simulink model "NumSim_standard_eVTOL"  (R2024b)
settings: Solver=ode14x  StartTime=0.0  StopTime=250  FixedStep=0.005  RelTol=1e-3
values from neighbouring files (symbols this model uses):
  aDl =     [initdata.mat]
  aDr =     [initdata.mat]
  aDyn =     [initdata.mat]
  Airport = init_airport('PHNL')    [initdata_HIL_eVTOL.m]
  aLat =     [initdata.mat]
  aLon =     [initdata.mat]
  D = Prop.D    [EOM_dt_MC.m]    (also in EOM_get_alf_dt_de_prop_evtol.m = CD * QS)
  dt0 = X(2)    [EOM_get_alf_dt_de_prop_evtol.m]    (also in initdata.mat = 0.258252593971; initdata_HIL_eVTOL.m = EOM_dt_MC)
  EAS0 = TAS0 / EAS2TAS    [initdata_HIL_eVTOL.m]
  FCS = init_FCS    [initdata_HIL_eVTOL.m]
  General = init_layoutdata    [EOM_dt_MC.m]    (also in build_optimized_CA.m; initdata.mat = ; initdata_HIL_eVTOL.m)
  h0 = Con(1)    [EOM_get_alf_dt_de_prop_evtol.m]    (also in initdata.mat = 450; initdata_HIL_eVTOL.m = 50)
  mass = Con(3)    [EOM_get_alf_dt_de_prop_evtol.m]    (also in initdata.mat = 2255.54; initdata_HIL_eVTOL.m = 7)
  Motor = init_motor_evtol    [EOM_dt_MC.m]    (also in initdata.mat = []; initdata_HIL_eVTOL.m)
  Prop = init_propeller_evtol_new    [EOM_dt_MC.m]    (also in initdata_HIL_eVTOL.m)
  R2D = 180/pi    (= 57.2957795131)    [EOM_get_alf_dt_de_prop_evtol.m]    (also in init_FCS.m; init_aerodata_evtol.m; init_airport.m; initdata.mat)
  theta0 = -0.0510981441662    [initdata.mat]
undefined symbols (not defined in the file or in its folder): A1, aDa, aDe, asbhl20env, B1, C1, de0, Earth, Environment, InitData, Kd, Kp, magnitude, Tc, WGS84
libraries: simulink_extras x26, simulink x18, slpidlib x14, vrlib x8, matrix_library x6, sharedutil x6, sharedtransform x5, aerolibwindfilters x4, aerolibatmos2 x3, aerolibobsolete x2, aerolibactuator x2, aerolibasang x2
(part 2 of 7)

== system NumSim_standard_eVTOL/FCS/FCS CMD ==
  note: FlightMod
      | 1-Ready
      | 2-TakeOff
      | 3-PullUp
      | 4-Climb
      | 5-Cruise, 5.1-circle, 5.2-line
      | 6-Return
      | 7-Approach
      | 8-Flare
      | 9-TouchDown
      | 10-Taxi
      | 11-GoAround
      | 12-Parachute
  note: LonMod:
      | 1-theta hold
      | 2-height hold
      | 3-gamma control
      | 4-landing flare control
      | 5-TakeOff
  note: LatMod:
      | 1-phi hold
      | 2-lateral deviation control
      | 3-taxi y control
      | 4-
      | 5-taxi y control
  note: VMod:
      | 1-cruise throt
      | 2-max throt
      | 3-min throt
      | 4-TECS
      | 5-Flare dt Fade
  SensorData : Inport
  Land_SW : Inport  Port=2
  Bus Creator1 : BusCreator  Inputs=14
  Bus Selector : BusSelector  OutputSignals=Xe,Va,Euler
  Clock : Clock
  Divide : Product  Inputs=*/
  Divide1 : Product  Inputs=**
  Gain : Gain  Gain=-1
  Ground : Ground
  ISA Atmosphere Model : aerolibatmos2/ISA Atmosphere Model  useExtended=off  action=Warning  custom=off  viscosityOut=off  g=9.80665  gamma=1.4  R=287.0531  L=0.0065  h_trop=11000  h_strat=20000  rho0=1.225  P0=101325  T0=288.15  h0=0  S=110.4  Tref=273.15  muref=1.716e-5
  Mode Generator : Stateflow chart  TreatAsAtomicUnit=on
  Rate Limiter : RateLimiter  RisingSlewLimit=5  FallingSlewLimit=-5  SampleTimeMode=inherited
  Scope : Scope
  Selector : Selector  InputPortWidth=3  IndexOptions=Index vector (dialog)  Indices=[1]  OutputSizes=1
  Selector1 : Selector  InputPortWidth=3  IndexOptions=Index vector (dialog)  Indices=2  OutputSizes=1
  Selector2 : Selector  InputPortWidth=3  IndexOptions=Index vector (dialog)  Indices=3  OutputSizes=1
  Selector3 : Selector  InputPortWidth=3  IndexOptions=Index vector (dialog)  Indices=3  OutputSizes=1
  Sqrt : Sqrt
  Terminator : Terminator
  Terminator1 : Terminator
  Terminator2 : Terminator
  hground_value : Constant  Value=Airport.Elevation_m  OutDataTypeStr=double
  phic1 : Constant  Value=1.225
  FCSCMD : Outport  VectorParamsAs1DForOutWhenUnconnected=off
  tag scope: icmd=global
  wires:
  [V] -> Mode Generator/3(V)
  [H] -> Mode Generator/1(H)
  Clock/1 -> Mode Generator/5(time)
  Mode Generator/12(L1mod) -> Bus Creator1/12  "L1Mod"
  Mode Generator/6(Vmod) -> Bus Creator1/6  "VMod"
  Mode Generator/2(Lonmod) -> Bus Creator1/2  "LonMod"
  Mode Generator/3(thetac) -> Bus Creator1/3  "thetac"
  Mode Generator/7(Vc) -> Divide1/1, Bus Creator1/7  "Vc_EAS"
  Mode Generator/8(Latmod) -> Bus Creator1/8  "LatMod"
  Mode Generator/4(gammac) -> Bus Creator1/4  "gammac"
  Mode Generator/9(phic) -> Bus Creator1/9  "phic"
  Mode Generator/11(yc) -> Bus Creator1/11  "yc"
  Mode Generator/10(chic) -> Bus Creator1/10  "chic"
  [x] -> Mode Generator/2(x)
  SensorData/1 -> Bus Selector/1
  Bus Selector/1 -> Selector/1, Selector1/1, Selector3/1  "<Xe>"
  Selector3/1 -> Gain/1
  Selector/1 -> [x]
  Gain/1 -> [H]
  Bus Selector/2 -> [V]  "<Va>"
  Ground/1 -> Mode Generator/6(psi0)
  Bus Selector/3 -> Selector2/1  "<Euler>"
  Selector2/1 -> [psi]
  Selector1/1 -> [y]
  hground_value/1 -> Mode Generator/4(h_runway)
  Mode Generator/1(FlightMod) -> Scope/1, Bus Creator1/1  "FlightMod"
  Bus Creator1/1 -> FCSCMD/1  "FCSCMD"
  [H] -> ISA Atmosphere Model/1
  ISA Atmosphere Model/4 -> Divide/2  "rho"
  phic1/1 -> Divide/1
  Divide/1 -> Sqrt/1
  Sqrt/1 -> Divide1/2
  Divide1/1 -> Bus Creator1/13  "Vc_TAS"
  ISA Atmosphere Model/1 -> Terminator/1
  ISA Atmosphere Model/2 -> Terminator1/1
  ISA Atmosphere Model/3 -> Terminator2/1
  Land_SW/1 -> Mode Generator/7(LAND_SW)
  Mode Generator/13(icmd) -> [icmd], Bus Creator1/14  "icmd"
  Mode Generator/5(hc) -> Rate Limiter/1  "Hc"
  Rate Limiter/1 -> Bus Creator1/5  "Hc"

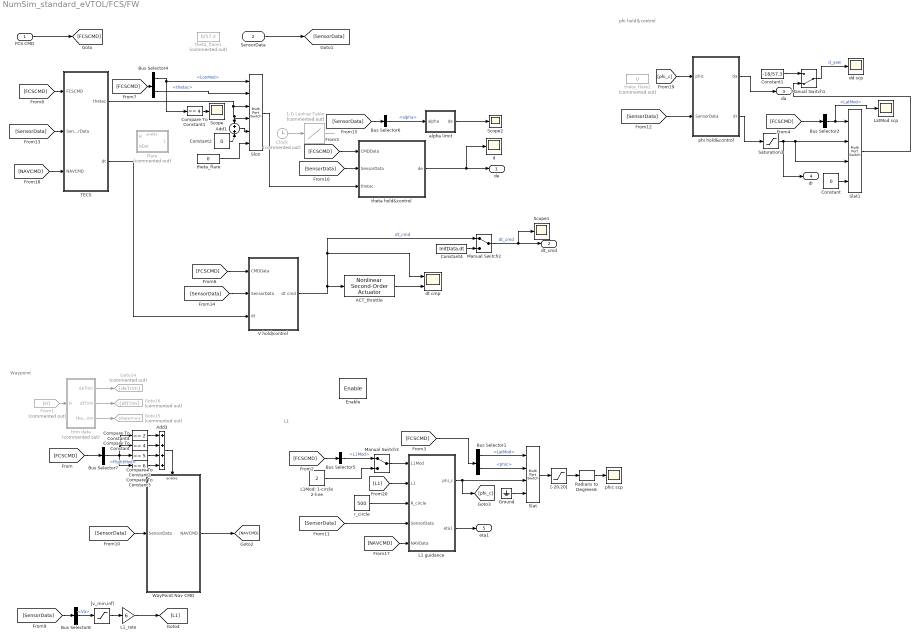
== system NumSim_standard_eVTOL/FCS/FW ==
  note: phi hold＆control
  note: L1
  note: Waypoint
  FCS CMD : Inport
  SensorData : Inport  Port=2
  Enable : EnablePort  StatesWhenEnabling=reset
  1-D Lookup Table : Lookup_n-D  Commented=on  NumberOfTableDimensions=1  BreakpointsForDimension1=[0,4,13,1e3]  Table=[-90,-90,0,0]./57.3  InternalRulePriority=Speed  RndMeth=Simplest
  ACT_throttle : aerolibactuator/Nonlinear Second-Order Actuator  wn_fin=50  z_fin=0.8  fin_max=FCS.dt_max  fin_min=FCS.dt_min  fin_maxrate=FCS.dt_rate  fin_act_0=InitData.dt  fin_act_vel=0
  Add1 : Sum  Inputs=+|+
  Add3 : Sum  Inputs=++++
  Bus Selector1 : BusSelector  OutputSignals=LatMod,phic
  Bus Selector2 : BusSelector  OutputSignals=LatMod
  Bus Selector4 : BusSelector  OutputSignals=LonMod,thetac
  Bus Selector5 : BusSelector  OutputSignals=L1Mod
  Bus Selector6 : BusSelector  OutputSignals=alpha
  Bus Selector7 : BusSelector  OutputSignals=FlightMod
  Bus Selector8 : BusSelector  OutputSignals=Va
  Clock : Clock  Commented=on
  Compare To Constant : simulink/Logic and Bit Operations/Compare To Constant  relop===  const=4  OutDataTypeStr=boolean
  Compare To Constant1 : simulink/Logic and Bit Operations/Compare To Constant  relop===  const=4  OutDataTypeStr=uint8  ZeroCross=off
  Compare To Constant2 : simulink/Logic and Bit Operations/Compare To Constant  relop===  const=5  OutDataTypeStr=boolean
  Compare To Constant3 : simulink/Logic and Bit Operations/Compare To Constant  relop===  const=6  OutDataTypeStr=boolean
  Compare To Constant4 : simulink/Logic and Bit Operations/Compare To Constant  relop===  const=2  OutDataTypeStr=boolean
  Constant : Constant  Value=0
  Constant1 : Constant  Value=-18/57.3
  Constant2 : Constant  Value=0
  Constant4 : Constant  Value=InitData.dt
  Flare : Subsystem  Commented=on
  From1 : From  Commented=on  GotoTag=H
      settings: CloseFcn=tagdialog Close
  Goto14 : Goto  Commented=on  GotoTag=deTrim  TagVisibility=scoped
  Goto15 : Goto  Commented=on  GotoTag=thetaTrim  TagVisibility=scoped
  Goto16 : Goto  Commented=on  GotoTag=dtTrim  TagVisibility=scoped
  Ground : Ground
  L1 guidance : Subsystem  RequirementInfo={} %GIDa_679a8677_8221_4c9e_b86c_be3e68c5d594
  L1Mod: 1-circle 2-line : Constant  Value=2
  L1_rate : Gain  Gain=6
  LatMod scp : Scope
  Manual Switch1 : ManualSwitch  CurrentSetting=0
  Manual Switch2 : ManualSwitch
  Manual Switch3 : ManualSwitch
  Radians to Degrees6 : simulink_extras/Transformations/Radians to Degrees
  Saturation3 : Saturate  UpperLimit=0.3  LowerLimit=-0.3
  Scope : Scope
  Scope1 : Scope
  Scope2 : Scope
  Slat : MultiPortSwitch  SaturateOnIntegerOverflow=off  InputSameDT=off
  Slat1 : MultiPortSwitch  SaturateOnIntegerOverflow=off  InputSameDT=off
  Slon : MultiPortSwitch  Inputs=5  DataPortIndices={2}  SaturateOnIntegerOverflow=off  InputSameDT=off
  TECS : Subsystem
  V hold/control : Subsystem
  WayPoint Nav CMD : Subsystem
  "[-20,20]" : Saturate  UpperLimit=20*pi/180  LowerLimit=-20*pi/180
  "[v_min,inf)" : Saturate  UpperLimit=inf  LowerLimit=FCS.V_min
  alpha limit : Subsystem
  d : Scope
  dd scp : Scope
  dt cmp : Scope  NumInputPorts=2
  phi hold&control : Subsystem
  phic scp : Scope
  r_circle : Constant  Value=500
  theta hold&control : Subsystem
  theta_flare : Constant  Value=0
  theta_flare1 : Constant  Commented=on  Value=0/57.3
  theta_flare2 : Constant  Commented=on  Value=0
  trim data : Subsystem  Commented=on
  de : Outport
  dt_cmd : Outport  Port=2
  da : Outport  Port=3
  dr : Outport  Port=4
  eta1 : Outport  Port=5
  wires:
  Compare To Constant4/1 -> Add3/1
  Bus Selector1/1 -> Slat/1  "<LatMod>"
  trim data/1(deTrim) -> Goto14/1
  WayPoint Nav CMD/1(NAVCMD) -> [NAVCMD]
  L1 guidance/2(eta1) -> eta1/1
  Slat/1 -> "[-20,20]"/1
  "[-20,20]"/1 -> Radians to Degrees6/1
  Add3/1 -> WayPoint Nav CMD/Enable
  r_circle/1 -> L1 guidance/3(R_circle)
  alpha limit/1(de) -> Scope2/1
  Ground/1 -> Slat/4
  V hold/control/1(dt cmd) -> Manual Switch2/1, dt cmp/1, ACT_throttle/1  "dt_cmd"
  L1Mod: 1-circle 2-line/1 -> Manual Switch3/2
  Constant4/1 -> Manual Switch2/2
  trim data/3(thetaTrim) -> Goto15/1
  ACT_throttle/1 -> dt cmp/2
  SensorData/1 -> [SensorData]
  Slat1/1 -> Manual Switch1/2
  Manual Switch1/1 -> dd scp/1  "d_yaw"
  Add1/1 -> Slon/5
  theta_flare/1 -> Slon/6
  Bus Selector2/1 -> LatMod scp/1, Slat1/1  "<LatMod>"
  Bus Selector5/1 -> Manual Switch3/1  "<L1Mod>"
  Bus Selector6/1 -> alpha limit/1(alpha)  "<alpha>"
  Bus Selector7/1 -> Compare To Constant3/1, Compare To Constant4/1, Compare To Constant/1, Compare To Constant2/1  "<FlightMod>"
  "[v_min,inf)"/1 -> L1_rate/1
  Clock/1 -> 1-D Lookup Table/1
  TECS/1(thetac) -> Add1/1, Slon/4, Slon/3
  Saturation3/1 -> dr/1, Slat1/3, Slat1/2
  Slon/1 -> theta hold&control/3(thetac)
  Bus Selector4/1 -> Compare To Constant1/1, Slon/1  "<LonMod>"
  1-D Lookup Table/1 -> ?
  TECS/2(dt) -> V hold/control/3(dt)
  Radians to Degrees6/1 -> phic scp/1
  Bus Selector4/2 -> Slon/2  "<thetac>"
  Bus Selector8/1 -> "[v_min,inf)"/1  "<Va>"
  From1/1 -> trim data/1(H)
  Manual Switch3/1 -> L1 guidance/1(L1Mod)
  phi hold&control/2(dr) -> Saturation3/1
  FCS CMD/1 -> [FCSCMD]
  Compare To Constant2/1 -> Add3/3
  Manual Switch2/1 -> Scope1/1, dt_cmd/1  "dt_cmd"
  Constant1/1 -> Manual Switch1/1
  Compare To Constant3/1 -> Add3/4
  trim data/2(dtTrim) -> Goto16/1
  Compare To Constant/1 -> Add3/2
  Bus Selector1/2 -> Slat/2  "<phic>"
  Constant2/1 -> Add1/2
  Constant/1 -> Slat1/4
  Compare To Constant1/1 -> Scope/1
  L1 guidance/1(phi_c) -> [phi_c], Slat/3
  theta hold&control/1(de) -> d/1, de/1
  phi hold&control/1(da) -> da/1
  [FCSCMD] -> Bus Selector7/1
  [FCSCMD] -> Bus Selector5/1
  [FCSCMD] -> Bus Selector1/1
  [FCSCMD] -> Bus Selector2/1
  [FCSCMD] -> theta hold&control/1(CMDData)
  [FCSCMD] -> V hold/control/1(CMDData)
  [FCSCMD] -> Bus Selector4/1
  [FCSCMD] -> TECS/1(FCSCMD)
  [SensorData] -> Bus Selector8/1
  [SensorData] -> WayPoint Nav CMD/1(SensorData)
  [SensorData] -> L1 guidance/4(SensorData)
  [SensorData] -> phi hold&control/2(SensorData)
  [SensorData] -> TECS/2(SensorData)
  [SensorData] -> V hold/control/2(SensorData)
  [SensorData] -> Bus Selector6/1
  [SensorData] -> theta hold&control/2(SensorData)
  [NAVCMD] -> L1 guidance/5(NAVData)
  [NAVCMD] -> TECS/3(NAVCMD)
  [phi_c] -> phi hold&control/1(phic)
  L1_rate/1 -> [L1]
  [L1] -> L1 guidance/2(L1)

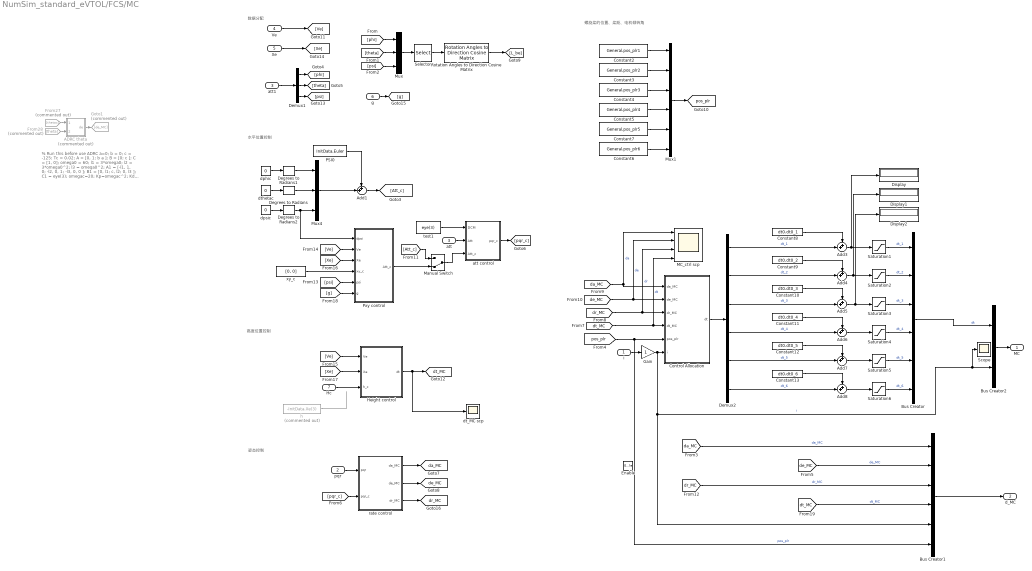
== system NumSim_standard_eVTOL/FCS/MC ==
  note: 数据分配
  note: 螺旋桨的位置、桨距、电机倾转角
  note: 姿态控制
  note: 高度位置控制
  note: 水平位置控制
  note: % Run this before use ADRC
      | a=0;
      | b = 0;
      | c = -125;
      | Tc = 0.02;
      | A = [0, 1; b a ];
      | B = [0; c ];
      | C = [1, 0];
      | omega0 = 60;
      | l1 = 3*omega0;
      | l2 = 3*omega0^2;
      | l3 = omega0^2;
      | A1 = [-l1,  1,  0; -l2,  0,  1; -l3,  0,  0 ];
      | B1 = [0,  l1; c,  l2; 0,  l3 ];
      | C1 = eye(3);
      | omegac=20;
      | Kp=omegac^2;
      | Kd = 2*omegac;
  i : Inport
  pqr : Inport  Port=2
  att : Inport  Port=3
  Ve : Inport  Port=4
  Xe : Inport  Port=5
  g : Inport  Port=6
  Hc : Inport  Port=7
  Enable : EnablePort  StatesWhenEnabling=reset
  ADRC theta : Subsystem  Commented=on
  Add{1,3..8} (7 alike) : Sum  Inputs=++|
  Bus Creator : BusCreator  Inputs=6
  Bus Creator1 : BusCreator  Inputs=6
  Bus Creator2 : BusCreator  Inputs=2
  Constant10 : Constant  Value=dt0.dt0_3
  Constant11 : Constant  Value=dt0.dt0_4
  Constant12 : Constant  Value=dt0.dt0_5
  Constant13 : Constant  Value=dt0.dt0_6
  Constant2 : Constant  Value=General.pos_plr1
  Constant3 : Constant  Value=General.pos_plr2
  Constant4 : Constant  Value=General.pos_plr3
  Constant5 : Constant  Value=General.pos_plr4
  Constant6 : Constant  Value=General.pos_plr6
  Constant7 : Constant  Value=General.pos_plr5
  Constant8 : Constant  Value=dt0.dt0_1
  Constant9 : Constant  Value=dt0.dt0_2
  Control Allocation : MATLAB Function  TreatAsAtomicUnit=on
  Degrees to Radians : simulink_extras/Transformations/Degrees to Radians
  Degrees to Radians1 : simulink_extras/Transformations/Degrees to Radians
  Degrees to Radians2 : simulink_extras/Transformations/Degrees to Radians
  Demux1 : Demux  Outputs=3
  Demux2 : Demux  Outputs=6
  Display : Display
  Display1 : Display
  Display2 : Display
  From27 : From  Commented=on  GotoTag=thetac
  From28 : From  Commented=on  GotoTag=theta
  Gain : Gain
  Goto1 : Goto  Commented=on  GotoTag=de_MC
  Height control : Subsystem
  MC_ctrl scp : Scope  NumInputPorts=4
  Manual Switch : ManualSwitch  CurrentSetting=0
  Mux : Mux  Inputs=3
  Mux1 : Mux  Inputs=6
  Mux4 : Mux  Inputs=3
  PSI0 : Constant  Value=InitData.Euler
  Pxy control : Subsystem
  Rotation Angles to Direction Cosine Matrix : sharedtransform/Rotation Angles to Direction Cosine Matrix  rotationOrder=ZYX  aMode=aMode
  Saturation{1..6} (6 alike) : Saturate  UpperLimit=1  LowerLimit=0
  Scope : Scope
  Selector : Selector  InputPortWidth=3  IndexOptions=Index vector (dialog)  Indices=[3,2,1]  OutputSizes=1
  att control : Subsystem
  att1 : InportShadow  Port=3
  dphic : Constant  Value=0
  dpsic : Constant  Value=0
  dt_MC scp : Scope
  dthetac : Constant  Value=0
  h : Constant  Commented=on  Value=-InitData.Xe(3)
  rate control : Subsystem
  test1 : Constant  Value=eye(3)
  xy_c : Constant  Value=[0, 0]
  MC : Outport
  d_MC : Outport  Port=2
  tag scope: da_MC=global, de_MC=global, dr_MC=global, dt_MC=global, pos_plr=global
  wires:
  Demux2/3 -> Add5/2  "dt_3"
  Demux2/2 -> Add4/2  "dt_2"
  Demux2/4 -> Add6/2  "dt_4"
  Demux2/1 -> Add3/2  "dt_1"
  Bus Creator/1 -> Bus Creator2/1  "dt"
  Rotation Angles to Direction Cosine Matrix/1 -> [L_be]
  Mux/1 -> Selector/1
  Selector/1 -> Rotation Angles to Direction Cosine Matrix/1
  [phi] -> Mux/1
  [psi] -> Mux/3
  Degrees to Radians/1 -> Mux4/2
  Degrees to Radians2/1 -> Pxy control/1(dpsi), Mux4/3
  [theta] -> Mux/2
  dphic/1 -> Degrees to Radians1/1
  dpsic/1 -> Degrees to Radians2/1
  Degrees to Radians1/1 -> Mux4/1
  [dt_MC] -> MC_ctrl scp/4, Control Allocation/4(dt_MC)  "dt"
  [da_MC] -> MC_ctrl scp/1, Control Allocation/1(da_MC)  "da"
  [de_MC] -> MC_ctrl scp/2, Control Allocation/2(de_MC)  "de"
  [dr_MC] -> MC_ctrl scp/3, Control Allocation/3(dr_MC)  "dr"
  From28/1 -> ADRC theta/2(theta)
  ADRC theta/1(de) -> Goto1/1
  From27/1 -> ADRC theta/1(thetac)
  pqr/1 -> rate control/1(pqr)
  [pqr_c] -> rate control/2(pqr_c)
  att/1 -> att control/2(Att)
  att control/1(pqr_c) -> [pqr_c]
  Mux4/1 -> Add1/2
  [Att_c] -> Manual Switch/1
  att1/1 -> Demux1/1
  Demux1/1 -> [phi]
  Demux1/3 -> [psi]
  Demux1/2 -> [theta]
  Ve/1 -> [Ve]
  Xe/1 -> [Xe]
  Pxy control/1(Att_c) -> Manual Switch/2
  xy_c/1 -> Pxy control/4(xy_c)
  Manual Switch/1 -> att control/3(Att_c)
  Add1/1 -> [Att_c]
  PSI0/1 -> Add1/1
  Control Allocation/1(dt) -> Demux2/1
  Height control/1(dt) -> dt_MC scp/1, [dt_MC]
  test1/1 -> att control/1(DCM)
  Hc/1 -> Height control/3(h_c)
  h/1 -> ?
  dthetac/1 -> Degrees to Radians/1
  Demux2/5 -> Add7/2  "dt_5"
  Demux2/6 -> Add8/2  "dt_6"
  rate control/1(da_MC) -> [da_MC]
  rate control/2(de_MC) -> [de_MC]
  rate control/3(dr_MC) -> [dr_MC]
  Constant2/1 -> Mux1/1
  Constant3/1 -> Mux1/2
  Constant4/1 -> Mux1/3
  Constant5/1 -> Mux1/4
  Constant7/1 -> Mux1/5
  Constant6/1 -> Mux1/6
  Mux1/1 -> [pos_plr]
  [pos_plr] -> Bus Creator1/6, Control Allocation/5(pos_plr)  "pos_plr"
  Gain/1 -> Scope/1, Bus Creator2/2, Bus Creator1/5, Control Allocation/6(i)  "i"
  Bus Creator2/1 -> MC/1
  Saturation1/1 -> Bus Creator/1  "dt_1"
  Saturation2/1 -> Bus Creator/2  "dt_2"
  Saturation3/1 -> Bus Creator/3  "dt_3"
  Saturation4/1 -> Bus Creator/4  "dt_4"
  Saturation5/1 -> Bus Creator/5  "dt_5"
  Saturation6/1 -> Bus Creator/6  "dt_6"
  Constant8/1 -> Add3/1
  Add3/1 -> Display/1, Saturation1/1
  Constant9/1 -> Add4/1
  Add4/1 -> Display1/1, Saturation2/1
  Constant10/1 -> Add5/1
  Add5/1 -> Display2/1, Saturation3/1
  Constant11/1 -> Add6/1
  Add6/1 -> Saturation4/1
  Constant12/1 -> Add7/1
  Add7/1 -> Saturation5/1
  Constant13/1 -> Add8/1
  Add8/1 -> Saturation6/1
  [psi] -> Pxy control/5(psi)
  [Ve] -> Pxy control/2(Ve)
  [Ve] -> Height control/1(Ve)
  [Xe] -> Pxy control/3(Xe)
  [Xe] -> Height control/2(Xe)
  g/1 -> [g]
  [g] -> Pxy control/6(g)
  i/1 -> Gain/1
  [de_MC] -> Bus Creator1/2  "de_MC"
  [dt_MC] -> Bus Creator1/4  "dt_MC"
  Bus Creator1/1 -> d_MC/1
  [da_MC] -> Bus Creator1/1  "da_MC"
  [dr_MC] -> Bus Creator1/3  "dr_MC"

== system NumSim_standard_eVTOL/FCS/control selector ==
  note: CtrlMod:
      | 1-pqr control
      | 2-att control
      | 3-path angle control
      | 4-way point control
      | 5-TakeOff
      | 6-Parachute land
  note: FlightStage
      | 1-Ready
      | 2-TakeOff
      | 3-PullUp
      | 4-Climb
      | 5-Cruise, 5.1-circle, 5.2-line
      | 6-Return
      | 7-Approach
      | 8-Flare
      | 9-TouchDown
      | 10-Taxi
      | 11-GoAround
      | 12-Parachute
  Bus Selector1 : BusSelector  Commented=on  OutputSignals=FlightMod
  Constant1 : Constant  Commented=on
  Constant8 : Constant  Commented=on  Value=0
  Constant9 : Constant  Commented=on
  From1 : From  Commented=on  GotoTag=CutAct
  From2 : From  Commented=on  GotoTag=CutAct
  From3 : From  Commented=on  GotoTag=CutAct
  From9 : From  Commented=on  GotoTag=deTrim  TagVisibility=scoped
      settings: CloseFcn=tagdialog Close
  Goto5 : Goto  Commented=on  GotoTag=CutAct
  Merge : Merge  Commented=on
  Product{,1..3} (4 alike) : Product  Commented=on
  Radians to Degrees1 : simulink_extras/Transformations/Radians to Degrees  Commented=on
  Scope : Scope  Commented=on
  Scope1 : Scope  Commented=on
  Switch Case : SwitchCase  Commented=on  CaseConditions={[2,12]}
  Switch Case Action Subsystem1 : Subsystem  Commented=on  TreatAsAtomicUnit=on
  Switch Case Action Subsystem2 : Subsystem  Commented=on  TreatAsAtomicUnit=on
  dr scp : Scope  Commented=on
  dt scp : Scope  Commented=on
  wires:
  Product/1 -> dt scp/1
  Switch Case Action Subsystem2/1(Out1) -> Merge/1
  Constant9/1 -> Switch Case Action Subsystem1/1(In1)  "keep"
  Switch Case Action Subsystem1/1(Out1) -> Merge/2
  Switch Case/1 -> Switch Case Action Subsystem2/Action
  Bus Selector1/1 -> Scope1/1, Switch Case/1  "<FlightMod>"
  Switch Case/2 -> Switch Case Action Subsystem1/Action
  Constant8/1 -> Switch Case Action Subsystem2/1(In1)  "cut"
  Merge/1 -> Goto5/1
  Constant1/1 -> Product/1
  From1/1 -> Product1/2
  From3/1 -> Product3/2
  From2/1 -> Product2/2
  Product2/1 -> dr scp/1
  Product1/1 -> Radians to Degrees1/1
  Radians to Degrees1/1 -> Scope/1
  ? -> ?

== system NumSim_standard_eVTOL/airframe/Flight Conditions ==
  EnvmData : Inport
  PlantData : Inport  Port=2
  Bus Selector1 : BusSelector  OutputSignals=WindVelocity,a,AirDensity,WindAngularRates,Po,To,g
  Bus Selector2 : BusSelector  OutputSignals=Ve,Vb,pqr,DCM_be
  Derivative : Derivative  CoefficientInTFapproximation=100
  Dynamic Pressure : aerolibasang/Dynamic Pressure
  "Incidence, Sideslip, & Airspeed" : Subsystem  AncestorBlock=aerolibasang/Incidence, Sideslip, & Airspeed  mask(Incidence,Sideslip,&Airspeed){}
      mask help: Calculate the angles between the body and the velocity vector (incidence and sideslip), and the velocity magnitude from the components in body axes (Vb).
      settings: LibrarySourceBlock=|
      | aerolibasang/Incidence, Sideslip,
      | & Airspeed
      mask Help: web(asbhelp('incidence'));
      mask Display:
      | port_label('input',1,'V_b','texmode','on');
      | port_label('output',1,'\alpha','texmode','on');
      | port_label('output',2,'\beta','texmode','on');
      | port_label('output',3,'V','texmode','on');
  Mach Number : aerolibasang/Mach Number
  Product : Product  Multiplication=Matrix(*)
  Product1 : Product  Multiplication=Matrix(*)
  Subsystem : Subsystem
  Sum1 : Sum  Inputs=+-|  InputSameDT=on  SaturateOnIntegerOverflow=on  OutDataTypeStr=Inherit: Same as first input
  Sum2 : Sum  Inputs=|+-  InputSameDT=on  SaturateOnIntegerOverflow=on  OutDataTypeStr=Inherit: Same as first input
  Terminator : Terminator
  Va_b : Scope
  Vk_b : Scope
  Vw_b : Scope
  Vw_e : Scope
  Alpha : Outport  VectorParamsAs1DForOutWhenUnconnected=off
  AlphaDot : Outport  Port=2  VectorParamsAs1DForOutWhenUnconnected=off
  Beta : Outport  Port=3  VectorParamsAs1DForOutWhenUnconnected=off
  V : Outport  Port=4  VectorParamsAs1DForOutWhenUnconnected=off
  pqrWind : Outport  Port=5  VectorParamsAs1DForOutWhenUnconnected=off
  Mach : Outport  Port=6  VectorParamsAs1DForOutWhenUnconnected=off
  Qbar : Outport  Port=7  InitialOutput=0  VectorParamsAs1DForOutWhenUnconnected=off
  gamma : Outport  Port=8  InitialOutput=0  VectorParamsAs1DForOutWhenUnconnected=off
  chi : Outport  Port=9  InitialOutput=0  VectorParamsAs1DForOutWhenUnconnected=off
  Po : Outport  Port=10  VectorParamsAs1DForOutWhenUnconnected=off
  To : Outport  Port=11  VectorParamsAs1DForOutWhenUnconnected=off
  g : Outport  Port=12  VectorParamsAs1DForOutWhenUnconnected=off
  wires:
  Derivative/1 -> AlphaDot/1
  Bus Selector1/4 -> Product1/2  "<WindAngularRates>"
  Subsystem/1(gamma) -> gamma/1
  PlantData/1 -> Bus Selector2/1
  Sum2/1 -> "Incidence, Sideslip, & Airspeed"/1(Vb), Va_b/1, Mach Number/1, Dynamic Pressure/1  "VA(b)"
  Subsystem/2(chi) -> chi/1
  Bus Selector2/2 -> Vk_b/1, Sum2/1  "<Vb>"
  Subsystem/3(V) -> Terminator/1
  Product1/1 -> Sum1/2
  Bus Selector1/5 -> Po/1  "<Po>"
  Mach Number/1 -> Mach/1  "Mach"
  "Incidence, Sideslip, & Airspeed"/1(Alpha) -> Derivative/1, Alpha/1  "Alpha"
  Product/1 -> Vw_b/1, Sum2/2
  Bus Selector2/1 -> Subsystem/1(<Ve>)  "<Ve>"
  "Incidence, Sideslip, & Airspeed"/2(Beta) -> Beta/1  "Beta"
  "Incidence, Sideslip, & Airspeed"/3(V) -> V/1  "V"
  Dynamic Pressure/1 -> Qbar/1  "qbar"
  Bus Selector1/2 -> Mach Number/2  "<a>"
  Bus Selector2/4 -> Product/1, Product1/1  "<DCM_be>"
  Bus Selector2/3 -> Sum1/1  "<pqr>"
  Sum1/1 -> pqrWind/1
  EnvmData/1 -> Bus Selector1/1
  Bus Selector1/3 -> Dynamic Pressure/2  "<AirDensity>"
  Bus Selector1/1 -> Product/2, Vw_e/1  "<WindVelocity>"
  Bus Selector1/7 -> g/1  "<g>"
  Bus Selector1/6 -> To/1  "<To>"

== system NumSim_standard_eVTOL/airframe/force moment ==
  note: force and moment in body fixed axis coordination
  PlantData : Inport
  Act_surface : Inport  Port=2
  prop : Inport  Port=3
  EnvmData : Inport  Port=4
  Add : Sum  Inputs=++++
  Add1 : Sum  Inputs=++++
  Disturbance : Constant  Value=[0,10,0]
  Disturbance1 : Constant  Value=[0,0,0]
  F_Gear_in_b scp : Scope  Commented=on
  Gear&FM in body axis : Subsystem  Commented=on
  M_Gear scp : Scope  Commented=on
  Manual Switch : ManualSwitch  CurrentSetting=0
  Motor moment scp : Scope
  Scope{,1..4,6} (6 alike) : Scope
  Thrust&M in body axis : Subsystem
  aero F&M in body axis : Subsystem
  gravity in body axis : Subsystem
  Fb (X Y Z) : Outport  VectorParamsAs1DForOutWhenUnconnected=off
  M (L M N) : Outport  Port=2  VectorParamsAs1DForOutWhenUnconnected=off
  wires:
  Thrust&M in body axis/1(f_T) -> Add/1, Scope4/1
  gravity in body axis/1(Fb) -> Add/3, Scope3/1
  Thrust&M in body axis/2(m_T) -> Add1/1, Motor moment scp/1
  aero F&M in body axis/2(M (L M N)) -> Scope6/1, Add1/2
  Add1/1 -> Scope1/1, M (L M N)/1
  Add/1 -> Scope/1, Fb (X Y Z)/1
  PlantData/1 -> aero F&M in body axis/1(PlantData), Gear&FM in body axis/1(PlantData), gravity in body axis/1(PlantData)
  Act_surface/1 -> aero F&M in body axis/2(Act_surface)
  EnvmData/1 -> gravity in body axis/2(EnvmData)
  Gear&FM in body axis/1(F_Gear) -> Add/4, F_Gear_in_b scp/1
  Gear&FM in body axis/2(M_Gear) -> Add1/3, M_Gear scp/1
  aero F&M in body axis/1(Fb (X Y Z)) -> Add/2, Scope2/1
  Disturbance/1 -> Manual Switch/1
  Manual Switch/1 -> Add1/4
  Disturbance1/1 -> Manual Switch/2
  prop/1 -> Thrust&M in body axis/1(prop)

== system NumSim_standard_eVTOL/Energy & Power/V_prop1/v_b to v_prop ==
  V_body : Inport
  i : Inport  Port=2
  Add : Sum  Inputs=+-
  Mux1 : Mux  Inputs=2
  Terminator : Terminator
  V_x : Fcn  Expr=u[1]*cos(u[4])
  V_y : Fcn  Expr=0
  V_z : Fcn  Expr=u[3]*sin(u[4])
  V : Outport  VectorParamsAs1DForOutWhenUnconnected=off
  wires:
  i/1 -> Mux1/2
  V_body/1 -> Mux1/1
  Mux1/1 -> V_z/1, V_y/1, V_x/1
  Add/1 -> V/1
  V_x/1 -> Add/1
  V_z/1 -> Add/2
  V_y/1 -> Terminator/1

== system NumSim_standard_eVTOL/Energy & Power/V_prop2/v_b to v_prop ==
  V_body : Inport
  i : Inport  Port=2
  Add : Sum  Inputs=+-
  Mux1 : Mux  Inputs=2
  Terminator : Terminator
  V_x : Fcn  Expr=u[1]*cos(u[4])
  V_y : Fcn  Expr=0
  V_z : Fcn  Expr=u[3]*sin(u[4])
  V : Outport  VectorParamsAs1DForOutWhenUnconnected=off
  wires:
  i/1 -> Mux1/2
  V_body/1 -> Mux1/1
  Mux1/1 -> V_z/1, V_y/1, V_x/1
  V_z/1 -> Add/2
  V_x/1 -> Add/1
  Add/1 -> V/1
  V_y/1 -> Terminator/1

== system NumSim_standard_eVTOL/Energy & Power/V_prop3/v_b to v_prop ==
  V_body : Inport
  i : Inport  Port=2
  Add : Sum  Inputs=+-
  Mux1 : Mux  Inputs=2
  Terminator : Terminator
  V_x : Fcn  Expr=u[1]*cos(u[4])
  V_y : Fcn  Expr=0
  V_z : Fcn  Expr=u[3]*sin(u[4])
  V : Outport  VectorParamsAs1DForOutWhenUnconnected=off
  wires:
  i/1 -> Mux1/2
  V_body/1 -> Mux1/1
  Mux1/1 -> V_z/1, V_y/1, V_x/1
  V_z/1 -> Add/2
  V_x/1 -> Add/1
  Add/1 -> V/1
  V_y/1 -> Terminator/1

== system NumSim_standard_eVTOL/Energy & Power/V_prop4/v_b to v_prop ==
  V_body : Inport
  i : Inport  Port=2
  Add : Sum  Inputs=+-
  Mux1 : Mux  Inputs=2
  Terminator : Terminator
  V_x : Fcn  Expr=u[1]*cos(u[4])
  V_y : Fcn  Expr=0
  V_z : Fcn  Expr=u[3]*sin(u[4])
  V : Outport  VectorParamsAs1DForOutWhenUnconnected=off
  wires:
  i/1 -> Mux1/2
  V_body/1 -> Mux1/1
  Mux1/1 -> V_z/1, V_y/1, V_x/1
  V_x/1 -> Add/1
  Add/1 -> V/1
  V_z/1 -> Add/2
  V_y/1 -> Terminator/1

== system NumSim_standard_eVTOL/Energy & Power/V_prop5/v_b to v_prop ==
  V_body : Inport
  i : Inport  Port=2
  Add : Sum  Inputs=+-
  Mux1 : Mux  Inputs=2
  Terminator : Terminator
  V_x : Fcn  Expr=u[1]*cos(u[4])
  V_y : Fcn  Expr=0
  V_z : Fcn  Expr=u[3]*sin(u[4])
  V : Outport  VectorParamsAs1DForOutWhenUnconnected=off
  wires:
  i/1 -> Mux1/2
  V_body/1 -> Mux1/1
  Mux1/1 -> V_z/1, V_y/1, V_x/1
  V_z/1 -> Add/2
  V_x/1 -> Add/1
  Add/1 -> V/1
  V_y/1 -> Terminator/1

== system NumSim_standard_eVTOL/Energy & Power/V_prop6/v_b to v_prop ==
  V_body : Inport
  i : Inport  Port=2
  Add : Sum  Inputs=+-
  Mux1 : Mux  Inputs=2
  Terminator : Terminator
  V_x : Fcn  Expr=u[1]*cos(u[4])
  V_y : Fcn  Expr=0
  V_z : Fcn  Expr=u[3]*sin(u[4])
  V : Outport  VectorParamsAs1DForOutWhenUnconnected=off
  wires:
  i/1 -> Mux1/2
  V_body/1 -> Mux1/1
  Mux1/1 -> V_z/1, V_y/1, V_x/1
  V_z/1 -> Add/2
  V_x/1 -> Add/1
  Add/1 -> V/1
  V_y/1 -> Terminator/1

== system NumSim_standard_eVTOL/Energy & Power/thrust_1/Motor ==
  P_shaft : Inport
  dt : Inport  Port=2
  V : Inport  Port=3
  rpm0 : Inport  Port=4
  rho : Inport  Port=5
  rpm_grid : Inport  Port=6
  Add : Sum
  Constant : Constant  Value=Motor.Ue
  Constant1 : Constant  Value=Motor.Re
  Constant2 : Constant  Value=Motor.Rm
  Constant3 : Constant  Value=Motor.KE
  Constant4 : Constant  Value=Motor.KT  VectorParams1D=off
  Constant5 : Constant  Value=Motor.Im0
  Constant6 : Constant  Value=0
  Constant7 : Constant  Value=0.001
  D^5 : Constant  Value=5
  Diameter : Constant  Value=Prop.D
  Diameter1 : Constant  Value=Prop.D
  Divide : Product  Inputs=*//
  Ea : Sum  Inputs=+-
  Gain1 : Gain  Gain=30/pi
  Gain2 : Gain  Gain=pi/30
  Gain3 : Gain  Gain=1/60
  Gain4 : Gain  Gain=1/(2*pi)
  Im : Sum
  Integrator : Integrator  InitialConditionSource=external  InitialCondition=600
  Ix : Constant  Value=Prop.Ix
  J : Product  Inputs=*//
  Manual Switch : ManualSwitch
  Math Function : Math  Operator=magnitude^2  SignedPower=on
  Math Function3 : Math  Operator=pow  SignedPower=on
  Math Function4 : Math  Operator=pow  SignedPower=on
  Memory : Memory  InitialCondition=0.1
  N(rpm) : Product  Inputs=*/
  N(rpm)1 : Product  Inputs=/*
  P Scope : Scope  NumInputPorts=2
  P_sp : Product  Inputs=4
  Product1 : Product
  Product2 : Product
  Q : Product  Inputs=4
  RPM 1 : Scope  NumInputPorts=2
  Saturation : Saturate  UpperLimit=1047.2  LowerLimit=0.1
  Scope : Scope
  Sum : Sum  Inputs=|+-
  Ueo : Product
  Um : Sum  Inputs=+-
  get CP : Lookup_n-D  BreakpointsForDimension1=Prop.J  BreakpointsForDimension2=Prop.rpm_grid  IndexSearchMethod=Linear search  BeginIndexSearchUsingPreviousIndexResult=on  Table=Prop.CP  RndMeth=Simplest
      settings: InputPortMap=u0,u1
  "n^3 " : Constant  Value=3
  rpm : Outport  VectorParamsAs1DForOutWhenUnconnected=off
  wires:
  Saturation/1 -> Gain1/1, Divide/2
  Gain2/1 -> Integrator/2
  rpm0/1 -> Manual Switch/1
  Gain1/1 -> rpm/1, RPM 1/1  "rpm"
  Sum/1 -> Divide/1  "DP"
  Divide/1 -> Integrator/1  "omega_dot"
  Integrator/1 -> Saturation/1  "omega"
  P_sp/1 -> Scope/1, P Scope/1, Sum/1
  P_shaft/1 -> P Scope/2, Sum/2
  Ix/1 -> Divide/3
  Constant/1 -> Ueo/2
  Ueo/1 -> Um/1
  Product1/1 -> Um/2
  Constant1/1 -> Product1/1
  Um/1 -> Ea/1
  Product2/1 -> Ea/2
  Constant2/1 -> Product2/1
  Ea/1 -> N(rpm)/1
  Constant3/1 -> N(rpm)/2
  Diameter/1 -> J/2
  V/1 -> J/1
  N(rpm)/1 -> Gain3/1, RPM 1/2
  J/1 -> get CP/1
  Gain4/1 -> Q/2  "CQ"
  D^5/1 -> Math Function4/2
  Diameter1/1 -> Math Function4/1
  Math Function/1 -> Q/3  "n^2"
  Q/1 -> N(rpm)1/2
  Constant4/1 -> N(rpm)1/1
  N(rpm)1/1 -> Im/1
  Constant5/1 -> Im/2
  Im/1 -> Product2/2, Product1/2
  rho/1 -> Q/1, P_sp/3  "rho"
  Math Function3/1 -> P_sp/2  "n^3"
  "n^3 "/1 -> Math Function3/2
  Math Function4/1 -> Q/4, P_sp/4  "D^5"
  get CP/1 -> P_sp/1, Gain4/1  "CP"
  Manual Switch/1 -> Gain2/1
  Constant6/1 -> Manual Switch/2
  Constant7/1 -> Add/1
  Add/1 -> Ueo/1
  dt/1 -> Add/2
  Gain3/1 -> Memory/1  "rps"
  Memory/1 -> J/3, Math Function3/1, Math Function/1
  rpm_grid/1 -> get CP/2

== system NumSim_standard_eVTOL/Energy & Power/thrust_1/Propeller  ==
  rpm : Inport
  V : Inport  Port=2
  rho : Inport  Port=3
  D^5 : Constant  Value=5
  Diameter : Constant  Value=Prop.D
  Display1 : Display
  Display7 : Display
  Divide : Product  Inputs=4
  Divide2 : Product  Inputs=4
  Divide3 : Product  Inputs=**/
  Gain : Gain  Gain=1/60
  Math Function : Math  Operator=magnitude^2  SignedPower=on
  Math Function1 : Math  Operator=magnitude^2  SignedPower=on
  Math Function2 : Math  Operator=magnitude^2  SignedPower=on
  Math Function3 : Math  Operator=pow  SignedPower=on
  Math Function4 : Math  Operator=pow  SignedPower=on
  Scope{,1..4} (5 alike) : Scope
  Subsystem : Subsystem
  get CP : Lookup_n-D  BreakpointsForDimension1=Prop.J  BreakpointsForDimension2=Prop.rpm_grid  IndexSearchMethod=Linear search  BeginIndexSearchUsingPreviousIndexResult=on  Table=Prop.CP  RndMeth=Simplest
      settings: InputPortMap=u0,u1
  get CT : Lookup_n-D  BreakpointsForDimension1=Prop.J  BreakpointsForDimension2=Prop.rpm_grid  IndexSearchMethod=Linear search  BeginIndexSearchUsingPreviousIndexResult=on  Table=Prop.CT  RndMeth=Simplest
      settings: InputPortMap=u0,u1
  "n^3 " : Constant  Value=3
  P_plr (w) : Outport  VectorParamsAs1DForOutWhenUnconnected=off
  T (N) : Outport  Port=2  VectorParamsAs1DForOutWhenUnconnected=off
  eta_p : Outport  Port=3  VectorParamsAs1DForOutWhenUnconnected=off
  wires:
  Divide2/1 -> Scope/1, P_plr (w)/1
  Divide3/1 -> eta_p/1  "eta_p"
  D^5/1 -> Math Function4/2
  Math Function4/1 -> Divide2/4
  "n^3 "/1 -> Math Function3/2
  Math Function3/1 -> Divide2/3
  get CP/1 -> Display1/1, Divide3/3, Divide2/1, Scope3/1
  rpm/1 -> get CP/2, get CT/2, Gain/1, Subsystem/2(rpm)
  Subsystem/1(J) -> Scope2/1, get CT/1, Divide3/1, get CP/1
  Divide/1 -> Scope1/1, T (N)/1
  Math Function2/1 -> Divide/4  "D^4"
  Math Function1/1 -> Math Function2/1
  Diameter/1 -> Math Function1/1, Math Function4/1
  Math Function/1 -> Divide/3  "n^2"
  Gain/1 -> Math Function3/1, Math Function/1
  rho/1 -> Divide/2, Divide2/2
  get CT/1 -> Display7/1, Divide3/2, Divide/1, Scope4/1
  V/1 -> Subsystem/1(V)

== system NumSim_standard_eVTOL/Energy & Power/thrust_2/Motor ==
  P_shaft : Inport
  dt : Inport  Port=2
  V : Inport  Port=3
  rpm0 : Inport  Port=4
  rho : Inport  Port=5
  rpm_grid : Inport  Port=6
  Constant : Constant  Value=Motor.Ue
  Constant1 : Constant  Value=Motor.Re
  Constant2 : Constant  Value=Motor.Rm
  Constant3 : Constant  Value=Motor.KE
  Constant4 : Constant  Value=Motor.KT  VectorParams1D=off
  Constant5 : Constant  Value=Motor.Im0
  Constant6 : Constant  Value=0
  D^5 : Constant  Value=5
  Diameter : Constant  Value=Prop.D
  Diameter1 : Constant  Value=Prop.D
  Divide : Product  Inputs=*//
  Ea : Sum  Inputs=+-
  Gain1 : Gain  Gain=30/pi
  Gain2 : Gain  Gain=pi/30
  Gain3 : Gain  Gain=1/60
  Gain4 : Gain  Gain=1/(2*pi)
  Im : Sum
  Integrator : Integrator  InitialConditionSource=external  InitialCondition=600
  Ix : Constant  Value=Prop.Ix
  J : Product  Inputs=*//
  Manual Switch : ManualSwitch
  Math Function : Math  Operator=magnitude^2  SignedPower=on
  Math Function3 : Math  Operator=pow  SignedPower=on
  Math Function4 : Math  Operator=pow  SignedPower=on
  Memory : Memory  InitialCondition=0.1
  N(rpm) : Product  Inputs=*/
  N(rpm)1 : Product  Inputs=/*
  P Scope : Scope  NumInputPorts=2
  P_sp : Product  Inputs=4
  Product1 : Product
  Product2 : Product
  Q : Product  Inputs=4
  RPM 2 : Scope
  Saturation : Saturate  UpperLimit=1047.2  LowerLimit=0.1
  Scope : Scope
  Sum : Sum  Inputs=|+-
  Ueo : Product
  Um : Sum  Inputs=+-
  get CP : Lookup_n-D  BreakpointsForDimension1=Prop.J  BreakpointsForDimension2=Prop.rpm_grid  IndexSearchMethod=Linear search  BeginIndexSearchUsingPreviousIndexResult=on  Table=Prop.CP  RndMeth=Simplest
      settings: InputPortMap=u0,u1
  "n^3 " : Constant  Value=3
  rpm : Outport  VectorParamsAs1DForOutWhenUnconnected=off
  wires:
  Saturation/1 -> Gain1/1, Divide/2
  Gain2/1 -> Integrator/2
  rpm0/1 -> Manual Switch/1
  Gain1/1 -> rpm/1, RPM 2/1  "rpm"
  Sum/1 -> Divide/1  "DP"
  Divide/1 -> Integrator/1  "omega_dot"
  dt/1 -> Ueo/1
  Integrator/1 -> Saturation/1  "omega"
  P_sp/1 -> Scope/1, P Scope/1, Sum/1
  P_shaft/1 -> P Scope/2, Sum/2
  Ix/1 -> Divide/3
  Constant/1 -> Ueo/2
  Ueo/1 -> Um/1
  Product1/1 -> Um/2
  Constant1/1 -> Product1/1
  Um/1 -> Ea/1
  Product2/1 -> Ea/2
  Constant2/1 -> Product2/1
  Ea/1 -> N(rpm)/1
  Constant3/1 -> N(rpm)/2
  Diameter/1 -> J/2
  V/1 -> J/1
  N(rpm)/1 -> Gain3/1
  J/1 -> get CP/1
  rpm_grid/1 -> get CP/2
  Gain4/1 -> Q/2  "CQ"
  D^5/1 -> Math Function4/2
  Diameter1/1 -> Math Function4/1
  Math Function/1 -> Q/3  "n^2"
  Q/1 -> N(rpm)1/2
  Constant4/1 -> N(rpm)1/1
  N(rpm)1/1 -> Im/1
  Constant5/1 -> Im/2
  Im/1 -> Product2/2, Product1/2
  rho/1 -> Q/1, P_sp/3  "rho"
  Math Function3/1 -> P_sp/2  "n^3"
  "n^3 "/1 -> Math Function3/2
  Math Function4/1 -> Q/4, P_sp/4  "D^5"
  get CP/1 -> Gain4/1, P_sp/1  "CP"
  Constant6/1 -> Manual Switch/2
  Manual Switch/1 -> Gain2/1
  Gain3/1 -> Memory/1  "rps"
  Memory/1 -> J/3, Math Function3/1, Math Function/1

== system NumSim_standard_eVTOL/Energy & Power/thrust_2/Propeller  ==
  rpm : Inport
  V : Inport  Port=2
  rho : Inport  Port=3
  D^5 : Constant  Value=5
  Diameter : Constant  Value=Prop.D
  Divide : Product  Inputs=4
  Divide2 : Product  Inputs=4
  Divide3 : Product  Inputs=**/
  Gain : Gain  Gain=1/60
  Math Function : Math  Operator=magnitude^2  SignedPower=on
  Math Function1 : Math  Operator=magnitude^2  SignedPower=on
  Math Function2 : Math  Operator=magnitude^2  SignedPower=on
  Math Function3 : Math  Operator=pow  SignedPower=on
  Math Function4 : Math  Operator=pow  SignedPower=on
  Scope{,1..4} (5 alike) : Scope
  Subsystem : Subsystem
  get CP : Lookup_n-D  BreakpointsForDimension1=Prop.J  BreakpointsForDimension2=Prop.rpm_grid  IndexSearchMethod=Linear search  BeginIndexSearchUsingPreviousIndexResult=on  Table=Prop.CP  RndMeth=Simplest
      settings: InputPortMap=u0,u1
  get CT : Lookup_n-D  BreakpointsForDimension1=Prop.J  BreakpointsForDimension2=Prop.rpm_grid  IndexSearchMethod=Linear search  BeginIndexSearchUsingPreviousIndexResult=on  Table=Prop.CT  RndMeth=Simplest
      settings: InputPortMap=u0,u1
  "n^3 " : Constant  Value=3
  P_plr (w) : Outport  VectorParamsAs1DForOutWhenUnconnected=off
  T (N) : Outport  Port=2  VectorParamsAs1DForOutWhenUnconnected=off
  eta_p : Outport  Port=3  VectorParamsAs1DForOutWhenUnconnected=off
  wires:
  Divide2/1 -> P_plr (w)/1, Scope/1
  Divide3/1 -> eta_p/1  "eta_p"
  D^5/1 -> Math Function4/2
  Math Function4/1 -> Divide2/4
  "n^3 "/1 -> Math Function3/2
  Math Function3/1 -> Divide2/3
  get CP/1 -> Divide3/3, Divide2/1, Scope3/1
  Subsystem/1(J) -> Scope2/1, get CT/1, Divide3/1, get CP/1
  Divide/1 -> Scope1/1, T (N)/1
  Math Function2/1 -> Divide/4  "D^4"
  Math Function1/1 -> Math Function2/1
  Diameter/1 -> Math Function1/1, Math Function4/1
  Math Function/1 -> Divide/3  "n^2"
  Gain/1 -> Math Function3/1, Math Function/1
  rho/1 -> Divide/2, Divide2/2
  get CT/1 -> Divide3/2, Divide/1, Scope4/1
  V/1 -> Subsystem/1(V)
  rpm/1 -> get CP/2, get CT/2, Gain/1, Subsystem/2(rpm)

== system NumSim_standard_eVTOL/Energy & Power/thrust_3/Motor ==
  P_shaft : Inport
  dt : Inport  Port=2
  V : Inport  Port=3
  rpm0 : Inport  Port=4
  rho : Inport  Port=5
  rpm_grid : Inport  Port=6
  Constant : Constant  Value=Motor.Ue
  Constant1 : Constant  Value=Motor.Re
  Constant2 : Constant  Value=Motor.Rm
  Constant3 : Constant  Value=Motor.KE
  Constant4 : Constant  Value=Motor.KT  VectorParams1D=off
  Constant5 : Constant  Value=Motor.Im0
  Constant6 : Constant  Value=0
  D^5 : Constant  Value=5
  Diameter : Constant  Value=Prop.D
  Diameter1 : Constant  Value=Prop.D
  Divide : Product  Inputs=*//
  Ea : Sum  Inputs=+-
  Gain1 : Gain  Gain=30/pi
  Gain2 : Gain  Gain=pi/30
  Gain3 : Gain  Gain=1/60
  Gain4 : Gain  Gain=1/(2*pi)
  Im : Sum
  Integrator : Integrator  InitialConditionSource=external  InitialCondition=600
  Ix : Constant  Value=Prop.Ix
  J : Product  Inputs=*//
  Manual Switch : ManualSwitch
  Math Function : Math  Operator=magnitude^2  SignedPower=on
  Math Function3 : Math  Operator=pow  SignedPower=on
  Math Function4 : Math  Operator=pow  SignedPower=on
  Memory : Memory  InitialCondition=0.1
  N(rpm) : Product  Inputs=*/
  N(rpm)1 : Product  Inputs=/*
  P Scope : Scope  NumInputPorts=2
  P_sp : Product  Inputs=4
  Product1 : Product
  Product2 : Product
  Q : Product  Inputs=4
  RPM 3 : Scope
  Saturation : Saturate  UpperLimit=1047.2  LowerLimit=0.1
  Scope : Scope
  Sum : Sum  Inputs=|+-
  Ueo : Product
  Um : Sum  Inputs=+-
  get CP : Lookup_n-D  BreakpointsForDimension1=Prop.J  BreakpointsForDimension2=Prop.rpm_grid  IndexSearchMethod=Linear search  BeginIndexSearchUsingPreviousIndexResult=on  Table=Prop.CP  RndMeth=Simplest
      settings: InputPortMap=u0,u1
  "n^3 " : Constant  Value=3
  rpm : Outport  VectorParamsAs1DForOutWhenUnconnected=off
  wires:
  Saturation/1 -> Gain1/1, Divide/2
  Gain2/1 -> Integrator/2
  rpm0/1 -> Manual Switch/1
  Gain1/1 -> rpm/1, RPM 3/1  "rpm"
  Sum/1 -> Divide/1  "DP"
  Divide/1 -> Integrator/1  "omega_dot"
  dt/1 -> Ueo/1
  Integrator/1 -> Saturation/1  "omega"
  P_sp/1 -> Scope/1, P Scope/1, Sum/1
  P_shaft/1 -> P Scope/2, Sum/2
  Ix/1 -> Divide/3
  Constant/1 -> Ueo/2
  Ueo/1 -> Um/1
  Product1/1 -> Um/2
  Constant1/1 -> Product1/1
  Um/1 -> Ea/1
  Product2/1 -> Ea/2
  Constant2/1 -> Product2/1
  Ea/1 -> N(rpm)/1
  Constant3/1 -> N(rpm)/2
  Diameter/1 -> J/2
  V/1 -> J/1
  N(rpm)/1 -> Gain3/1
  J/1 -> get CP/1
  rpm_grid/1 -> get CP/2
  Gain4/1 -> Q/2  "CQ"
  D^5/1 -> Math Function4/2
  Diameter1/1 -> Math Function4/1
  Math Function/1 -> Q/3  "n^2"
  Q/1 -> N(rpm)1/2
  Constant4/1 -> N(rpm)1/1
  N(rpm)1/1 -> Im/1
  Constant5/1 -> Im/2
  Im/1 -> Product1/2, Product2/2
  rho/1 -> Q/1, P_sp/3  "rho"
  Math Function3/1 -> P_sp/2  "n^3"
  "n^3 "/1 -> Math Function3/2
  Math Function4/1 -> Q/4, P_sp/4  "D^5"
  get CP/1 -> Gain4/1, P_sp/1  "CP"
  Constant6/1 -> Manual Switch/2
  Manual Switch/1 -> Gain2/1
  Gain3/1 -> Memory/1  "rps"
  Memory/1 -> J/3, Math Function3/1, Math Function/1

== system NumSim_standard_eVTOL/Energy & Power/thrust_3/Propeller  ==
  rpm : Inport
  V : Inport  Port=2
  rho : Inport  Port=3
  D^5 : Constant  Value=5
  Diameter : Constant  Value=Prop.D
  Divide : Product  Inputs=4
  Divide2 : Product  Inputs=4
  Divide3 : Product  Inputs=**/
  Gain : Gain  Gain=1/60
  Math Function : Math  Operator=magnitude^2  SignedPower=on
  Math Function1 : Math  Operator=magnitude^2  SignedPower=on
  Math Function2 : Math  Operator=magnitude^2  SignedPower=on
  Math Function3 : Math  Operator=pow  SignedPower=on
  Math Function4 : Math  Operator=pow  SignedPower=on
  Scope{,1..4} (5 alike) : Scope
  Subsystem : Subsystem
  get CP : Lookup_n-D  BreakpointsForDimension1=Prop.J  BreakpointsForDimension2=Prop.rpm_grid  IndexSearchMethod=Linear search  BeginIndexSearchUsingPreviousIndexResult=on  Table=Prop.CP  RndMeth=Simplest
      settings: InputPortMap=u0,u1
  get CT : Lookup_n-D  BreakpointsForDimension1=Prop.J  BreakpointsForDimension2=Prop.rpm_grid  IndexSearchMethod=Linear search  BeginIndexSearchUsingPreviousIndexResult=on  Table=Prop.CT  RndMeth=Simplest
      settings: InputPortMap=u0,u1
  "n^3 " : Constant  Value=3
  P_plr (w) : Outport  VectorParamsAs1DForOutWhenUnconnected=off
  T (N) : Outport  Port=2  VectorParamsAs1DForOutWhenUnconnected=off
  eta_p : Outport  Port=3  VectorParamsAs1DForOutWhenUnconnected=off
  wires:
  Divide2/1 -> P_plr (w)/1, Scope/1
  Divide3/1 -> eta_p/1  "eta_p"
  D^5/1 -> Math Function4/2
  Math Function4/1 -> Divide2/4
  "n^3 "/1 -> Math Function3/2
  Math Function3/1 -> Divide2/3
  get CP/1 -> Divide3/3, Divide2/1, Scope3/1
  Subsystem/1(J) -> Scope2/1, get CT/1, Divide3/1, get CP/1
  Divide/1 -> Scope1/1, T (N)/1
  Math Function2/1 -> Divide/4  "D^4"
  Math Function1/1 -> Math Function2/1
  Diameter/1 -> Math Function1/1, Math Function4/1
  Math Function/1 -> Divide/3  "n^2"
  Gain/1 -> Math Function3/1, Math Function/1
  rho/1 -> Divide/2, Divide2/2
  get CT/1 -> Divide3/2, Divide/1, Scope4/1
  V/1 -> Subsystem/1(V)
  rpm/1 -> get CP/2, get CT/2, Gain/1, Subsystem/2(rpm)

== system NumSim_standard_eVTOL/Energy & Power/thrust_4/Motor ==
  P_shaft : Inport
  dt : Inport  Port=2
  V : Inport  Port=3
  rpm0 : Inport  Port=4
  rho : Inport  Port=5
  rpm_grid : Inport  Port=6
  Constant : Constant  Value=Motor.Ue
  Constant1 : Constant  Value=Motor.Re
  Constant2 : Constant  Value=Motor.Rm
  Constant3 : Constant  Value=Motor.KE
  Constant4 : Constant  Value=Motor.KT  VectorParams1D=off
  Constant5 : Constant  Value=Motor.Im0
  Constant6 : Constant  Value=0
  D^5 : Constant  Value=5
  Diameter : Constant  Value=Prop.D
  Diameter1 : Constant  Value=Prop.D
  Divide : Product  Inputs=*//
  Ea : Sum  Inputs=+-
  Gain1 : Gain  Gain=30/pi
  Gain2 : Gain  Gain=pi/30
  Gain3 : Gain  Gain=1/60
  Gain4 : Gain  Gain=1/(2*pi)
  Im : Sum
  Integrator : Integrator  InitialConditionSource=external  InitialCondition=600
  Ix : Constant  Value=Prop.Ix
  J : Product  Inputs=*//
  Manual Switch : ManualSwitch
  Math Function : Math  Operator=magnitude^2  SignedPower=on
  Math Function3 : Math  Operator=pow  SignedPower=on
  Math Function4 : Math  Operator=pow  SignedPower=on
  Memory : Memory  InitialCondition=0.1
  N(rpm) : Product  Inputs=*/
  N(rpm)1 : Product  Inputs=/*
  P Scope : Scope  NumInputPorts=2
  P_sp : Product  Inputs=4
  Product1 : Product
  Product2 : Product
  Q : Product  Inputs=4
  RPM 4 : Scope  NumInputPorts=2
  Saturation : Saturate  UpperLimit=1047.2  LowerLimit=0.1
  Scope : Scope
  Scope1 : Scope
  Scope2 : Scope
  Sum : Sum  Inputs=|+-
  Ueo : Product
  Um : Sum  Inputs=+-
  get CP : Lookup_n-D  BreakpointsForDimension1=Prop.J  BreakpointsForDimension2=Prop.rpm_grid  IndexSearchMethod=Linear search  BeginIndexSearchUsingPreviousIndexResult=on  Table=Prop.CP  RndMeth=Simplest
      settings: InputPortMap=u0,u1
  "n^3 " : Constant  Value=3
  rpm : Outport  VectorParamsAs1DForOutWhenUnconnected=off
  wires:
  Saturation/1 -> Gain1/1, Divide/2
  Gain2/1 -> Integrator/2
  rpm0/1 -> Manual Switch/1
  Gain1/1 -> rpm/1, RPM 4/1  "rpm"
  Sum/1 -> Divide/1  "DP"
  Divide/1 -> Integrator/1  "omega_dot"
  dt/1 -> Ueo/1
  Integrator/1 -> Saturation/1  "omega"
  P_sp/1 -> Scope/1, P Scope/1, Sum/1
  P_shaft/1 -> P Scope/2, Sum/2
  Ix/1 -> Divide/3
  Constant/1 -> Ueo/2
  Ueo/1 -> Um/1
  Product1/1 -> Um/2
  Constant1/1 -> Product1/1
  Um/1 -> Ea/1
  Product2/1 -> Ea/2
  Constant2/1 -> Product2/1
  Ea/1 -> N(rpm)/1
  Constant3/1 -> N(rpm)/2
  Diameter/1 -> J/2
  V/1 -> J/1
  N(rpm)/1 -> Gain3/1, RPM 4/2
  J/1 -> Scope1/1, get CP/1
  rpm_grid/1 -> get CP/2
  Gain4/1 -> Q/2  "CQ"
  D^5/1 -> Math Function4/2
  Diameter1/1 -> Math Function4/1
  Math Function/1 -> Q/3  "n^2"
  Q/1 -> N(rpm)1/2
  Constant4/1 -> N(rpm)1/1
  N(rpm)1/1 -> Im/1
  Constant5/1 -> Im/2
  Im/1 -> Product1/2, Product2/2
  rho/1 -> Q/1, P_sp/3  "rho"
  Math Function3/1 -> P_sp/2  "n^3"
  "n^3 "/1 -> Math Function3/2
  Math Function4/1 -> Q/4, P_sp/4  "D^5"
  get CP/1 -> Gain4/1, Scope2/1, P_sp/1  "CP"
  Constant6/1 -> Manual Switch/2
  Manual Switch/1 -> Gain2/1
  Gain3/1 -> Memory/1
  Memory/1 -> J/3, Math Function3/1, Math Function/1

== system NumSim_standard_eVTOL/Energy & Power/thrust_4/Propeller  ==
  rpm : Inport
  V : Inport  Port=2
  rho : Inport  Port=3
  D^5 : Constant  Value=5
  Diameter : Constant  Value=Prop.D
  Divide : Product  Inputs=4
  Divide2 : Product  Inputs=4
  Divide3 : Product  Inputs=**/
  Gain : Gain  Gain=1/60
  Math Function : Math  Operator=magnitude^2  SignedPower=on
  Math Function1 : Math  Operator=magnitude^2  SignedPower=on
  Math Function2 : Math  Operator=magnitude^2  SignedPower=on
  Math Function3 : Math  Operator=pow  SignedPower=on
  Math Function4 : Math  Operator=pow  SignedPower=on
  Scope{,1..4} (5 alike) : Scope
  Subsystem : Subsystem
  get CP : Lookup_n-D  BreakpointsForDimension1=Prop.J  BreakpointsForDimension2=Prop.rpm_grid  IndexSearchMethod=Linear search  BeginIndexSearchUsingPreviousIndexResult=on  Table=Prop.CP  RndMeth=Simplest
      settings: InputPortMap=u0,u1
  get CT : Lookup_n-D  BreakpointsForDimension1=Prop.J  BreakpointsForDimension2=Prop.rpm_grid  IndexSearchMethod=Linear search  BeginIndexSearchUsingPreviousIndexResult=on  Table=Prop.CT  RndMeth=Simplest
      settings: InputPortMap=u0,u1
  "n^3 " : Constant  Value=3
  P_plr (w) : Outport  VectorParamsAs1DForOutWhenUnconnected=off
  T (N) : Outport  Port=2  VectorParamsAs1DForOutWhenUnconnected=off
  eta_p : Outport  Port=3  VectorParamsAs1DForOutWhenUnconnected=off
  wires:
  Divide2/1 -> P_plr (w)/1, Scope/1
  Divide3/1 -> eta_p/1  "eta_p"
  D^5/1 -> Math Function4/2
  Math Function4/1 -> Divide2/4
  "n^3 "/1 -> Math Function3/2
  Math Function3/1 -> Divide2/3
  get CP/1 -> Divide3/3, Divide2/1, Scope3/1
  Subsystem/1(J) -> Scope2/1, get CT/1, Divide3/1, get CP/1
  Divide/1 -> Scope1/1, T (N)/1
  Math Function2/1 -> Divide/4  "D^4"
  Math Function1/1 -> Math Function2/1
  Diameter/1 -> Math Function1/1, Math Function4/1
  Math Function/1 -> Divide/3  "n^2"
  Gain/1 -> Math Function3/1, Math Function/1
  rho/1 -> Divide/2, Divide2/2
  get CT/1 -> Divide3/2, Divide/1, Scope4/1
  V/1 -> Subsystem/1(V)
  rpm/1 -> get CP/2, get CT/2, Gain/1, Subsystem/2(rpm)
